simulink library "nsd"  (Simulink 8.1)
settings: Solver=ode1  StartTime=0.0  StopTime=Inf  FixedStep=0.001  RelTol=1e-3
PostLoadFcn:
  | , if any(exist('dsrtsu_mdlpostloadfcn', 'file') == [2, 3, 6]), try dsrtsu_mdlpostloadfcn('Execute', bdroot); catch fprintf('Error in PostLoadFcn (dsrtsu_mdlpostloadfcn) for model "%s":\n %s\n', bdroot, lasterr); end, end,
undefined symbols (not defined in the file or in its folder): KIFO_SameDirecSpeed_kph
libraries: hcu_lib x1
settings Model: DSRTSU_INTERNAL_RTI_VER=450  DSRTSU_INTERNAL_RTI_TYPE=rti1401  RTICANMMDATA=struct('GeneralSetupData',struct('modelroot','D:\ELN150201\Phase3\branches\Model_with_Distance_trigger\AdasDragon\software\sw_development\arch\app\ifo','generalsettings',struct('filesettings',struct('destfolder',struct('Name','RTICANMM_FILES','Check',1),'buildfolder',struct('Name','.','Check',1),'AbsDestfolder',struct('Name','D:\ELN150201\Phase3\branches\Model_with_Distance_trigger\AdasDragon\software\sw_development\arch\app\ifo\RTICANMM_FILES'),'AbsBuildfolder',struct('Name','D:\ELN150201\Phase3\branches\Model_with_Distance_trigger\AdasDragon\software\sw_development\arch\app\ifo'))),'options',struct('addpaths',1,'rmpaths',1,'addtrcexclusion',logical(1),'cannavigator',struct('checkmonitoring',0),'show_usrtrc',0,'use_usrtrc',0),'advanced',struct('options',[1 1 1 1 1 1 1 1 1 1 1 1 1 1 1 1 1 1 1 1 1 1 1 1 1 1 1 1 1 1 1 1 1 1 1 1 1 1 1 1 1 1 1 1 1 1 1 1 1 1 1 1 1 1 1 1 1 1 1 1 1 1 1 1 1 1 1 1 1 1 1 1 1 1 1 1 1 1 1 1 1 1 1 1 1 1 1 1 1 1 1 1 1 1 1 1 1 1 1 1]),'MPSetup',{{}},'modelname','nsd','block','nsd'))  DSRTSU_INTERNAL_RTIFPGA=40  Creator=tescamilla  LastModifiedBy=AT015555

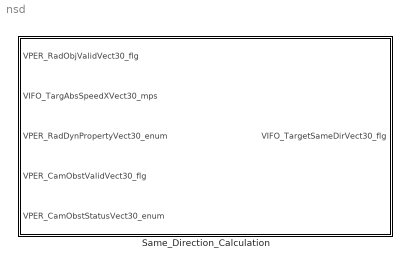
== system nsd ==
  Same_Direction_Calculation : Subsystem

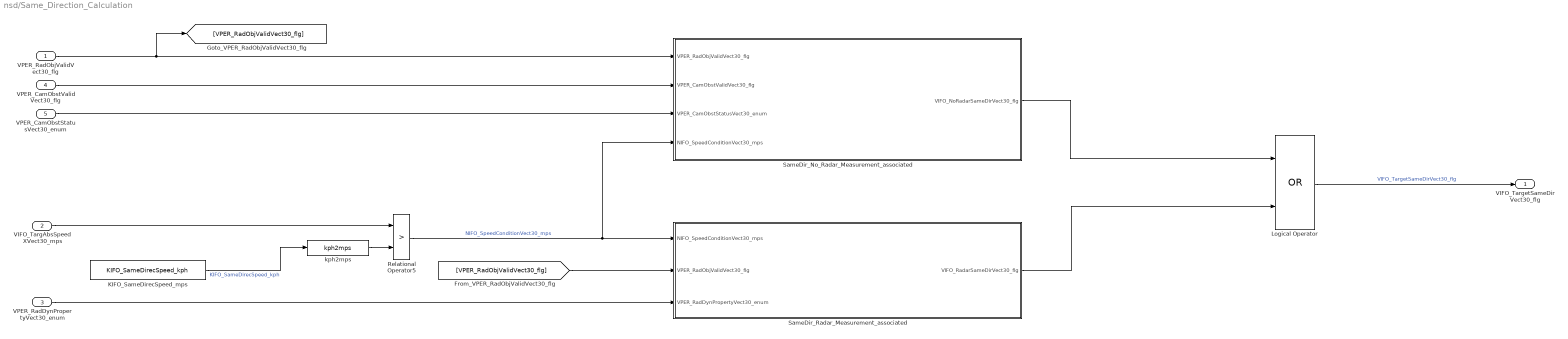
== system nsd/Same_Direction_Calculation ==
  VPER_RadObjValidVect30_flg : Inport
  VIFO_TargAbsSpeedXVect30_mps : Inport  Port=2
  VPER_RadDynPropertyVect30_enum : Inport  Port=3
  VPER_CamObstValidVect30_flg : Inport  Port=4
  VPER_CamObstStatusVect30_enum : Inport  Port=5
  KIFO_SameDirecSpeed_mps : Constant  Value=KIFO_SameDirecSpeed_kph  OutDataTypeStr=single
  Logical Operator : Logic  Operator=OR  AllPortsSameDT=off  OutDataTypeStr=boolean
  Relational Operator5 : RelationalOperator  Operator=>  OutDataTypeStr=boolean
  SameDir_No_Radar_Measurement_associated : Subsystem  TreatAsAtomicUnit=on
  SameDir_Radar_Measurement_associated : Subsystem  TreatAsAtomicUnit=on
  kph2mps : hcu_lib/kph2mps
  VIFO_TargetSameDirVect30_flg : Outport
  wires:
  Logical Operator/1 -> VIFO_TargetSameDirVect30_flg/1  "VIFO_TargetSameDirVect30_flg"
  VIFO_TargAbsSpeedXVect30_mps/1 -> Relational Operator5/1
  KIFO_SameDirecSpeed_mps/1 -> kph2mps/1  "KIFO_SameDirecSpeed_kph"
  kph2mps/1 -> Relational Operator5/2
  Relational Operator5/1 -> SameDir_No_Radar_Measurement_associated/4(NIFO_SpeedConditionVect30_mps), SameDir_Radar_Measurement_associated/1(NIFO_SpeedConditionVect30_mps)  "NIFO_SpeedConditionVect30_mps"
  SameDir_No_Radar_Measurement_associated/1(VIFO_NoRadarSameDirVect30_flg) -> Logical Operator/1
  SameDir_Radar_Measurement_associated/1(VIFO_RadarSameDirVect30_flg) -> Logical Operator/2
  VPER_RadObjValidVect30_flg/1 -> [VPER_RadObjValidVect30_flg], SameDir_No_Radar_Measurement_associated/1(VPER_RadObjValidVect30_flg)
  VPER_CamObstValidVect30_flg/1 -> SameDir_No_Radar_Measurement_associated/2(VPER_CamObstValidVect30_flg)
  VPER_CamObstStatusVect30_enum/1 -> SameDir_No_Radar_Measurement_associated/3(VPER_CamObstStatusVect30_enum)
  VPER_RadDynPropertyVect30_enum/1 -> SameDir_Radar_Measurement_associated/3(VPER_RadDynPropertyVect30_enum)
  [VPER_RadObjValidVect30_flg] -> SameDir_Radar_Measurement_associated/2(VPER_RadObjValidVect30_flg)

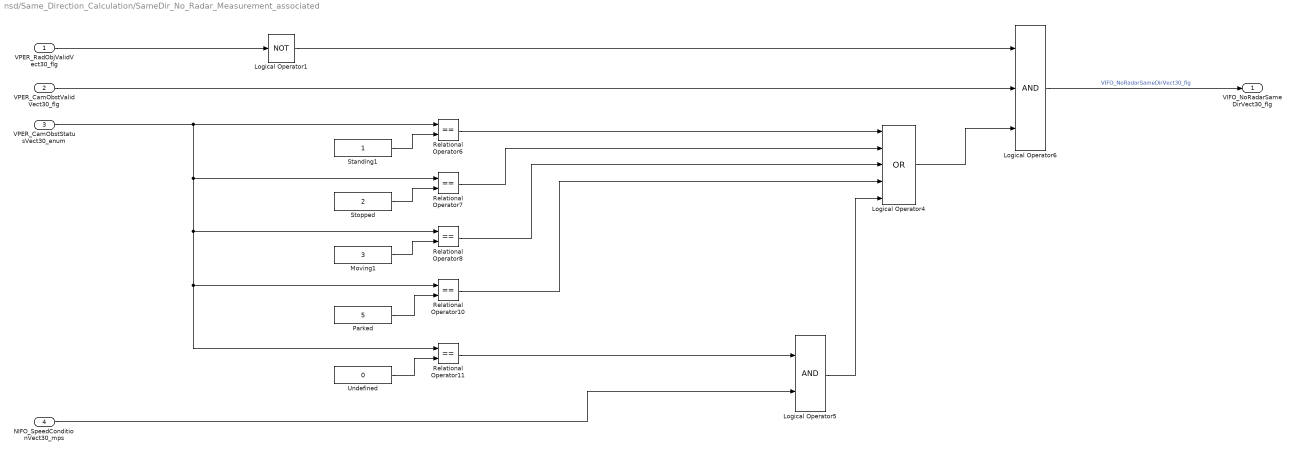
== system nsd/Same_Direction_Calculation/SameDir_No_Radar_Measurement_associated ==
  VPER_RadObjValidVect30_flg : Inport
  VPER_CamObstValidVect30_flg : Inport  Port=2
  VPER_CamObstStatusVect30_enum : Inport  Port=3
  NIFO_SpeedConditionVect30_mps : Inport  Port=4
  Logical Operator1 : Logic  Operator=NOT  AllPortsSameDT=off  OutDataTypeStr=boolean
  Logical Operator4 : Logic  Operator=OR  Inputs=5  AllPortsSameDT=off  OutDataTypeStr=boolean
  Logical Operator5 : Logic  AllPortsSameDT=off  OutDataTypeStr=boolean
  Logical Operator6 : Logic  Inputs=3  AllPortsSameDT=off  OutDataTypeStr=boolean
  Moving1 : Constant  Value=3
  Parked : Constant  Value=5
  Relational Operator{6..8,10..11} (5 alike) : RelationalOperator  Operator===  OutDataTypeStr=boolean
  Standing1 : Constant
  Stopped : Constant  Value=2
  Undefined : Constant  Value=0
  VIFO_NoRadarSameDirVect30_flg : Outport
  wires:
  Standing1/1 -> Relational Operator6/2
  Stopped/1 -> Relational Operator7/2
  Moving1/1 -> Relational Operator8/2
  Parked/1 -> Relational Operator10/2
  Relational Operator6/1 -> Logical Operator4/1
  Relational Operator7/1 -> Logical Operator4/2
  Relational Operator8/1 -> Logical Operator4/3
  Relational Operator10/1 -> Logical Operator4/4
  Undefined/1 -> Relational Operator11/2
  VPER_CamObstStatusVect30_enum/1 -> Relational Operator11/1, Relational Operator10/1, Relational Operator8/1, Relational Operator7/1, Relational Operator6/1
  Relational Operator11/1 -> Logical Operator5/1
  NIFO_SpeedConditionVect30_mps/1 -> Logical Operator5/2
  Logical Operator5/1 -> Logical Operator4/5
  VPER_CamObstValidVect30_flg/1 -> Logical Operator6/2
  Logical Operator4/1 -> Logical Operator6/3
  Logical Operator6/1 -> VIFO_NoRadarSameDirVect30_flg/1  "VIFO_NoRadarSameDirVect30_flg"
  VPER_RadObjValidVect30_flg/1 -> Logical Operator1/1
  Logical Operator1/1 -> Logical Operator6/1

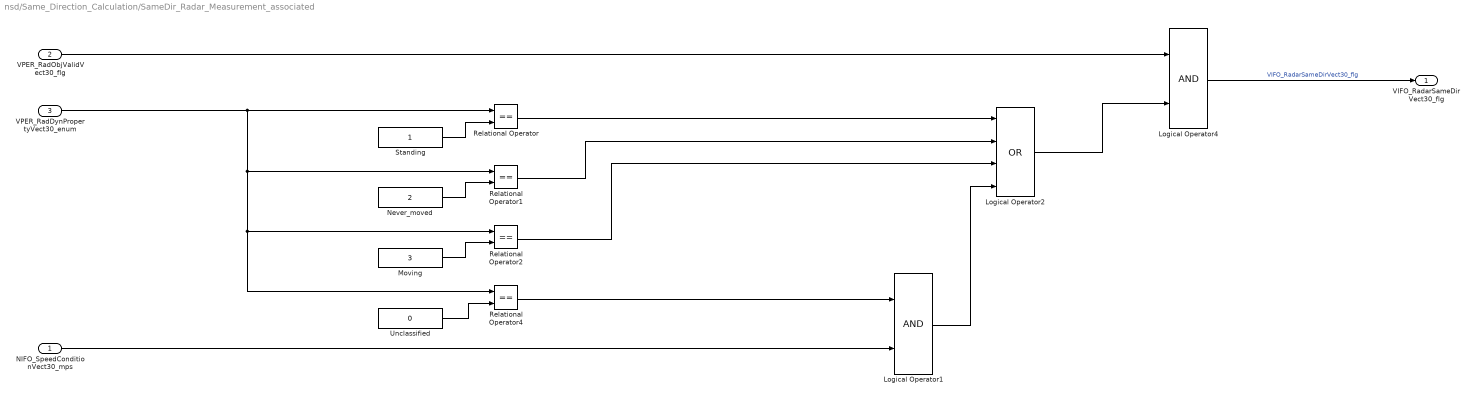
== system nsd/Same_Direction_Calculation/SameDir_Radar_Measurement_associated ==
  NIFO_SpeedConditionVect30_mps : Inport
  VPER_RadObjValidVect30_flg : Inport  Port=2
  VPER_RadDynPropertyVect30_enum : Inport  Port=3
  Logical Operator1 : Logic  AllPortsSameDT=off  OutDataTypeStr=boolean
  Logical Operator2 : Logic  Operator=OR  Inputs=4  AllPortsSameDT=off  OutDataTypeStr=boolean
  Logical Operator4 : Logic  AllPortsSameDT=off  OutDataTypeStr=boolean
  Moving : Constant  Value=3
  Never_moved : Constant  Value=2
  Relational Operator{,1..2,4} (4 alike) : RelationalOperator  Operator===  OutDataTypeStr=boolean
  Standing : Constant
  Unclassified : Constant  Value=0
  VIFO_RadarSameDirVect30_flg : Outport
  wires:
  Standing/1 -> Relational Operator/2
  Never_moved/1 -> Relational Operator1/2
  Moving/1 -> Relational Operator2/2
  Unclassified/1 -> Relational Operator4/2
  VPER_RadDynPropertyVect30_enum/1 -> Relational Operator4/1, Relational Operator2/1, Relational Operator1/1, Relational Operator/1
  Relational Operator/1 -> Logical Operator2/1
  Relational Operator1/1 -> Logical Operator2/2
  Relational Operator2/1 -> Logical Operator2/3
  Relational Operator4/1 -> Logical Operator1/1
  NIFO_SpeedConditionVect30_mps/1 -> Logical Operator1/2
  Logical Operator1/1 -> Logical Operator2/4
  Logical Operator2/1 -> Logical Operator4/2
  VPER_RadObjValidVect30_flg/1 -> Logical Operator4/1
  Logical Operator4/1 -> VIFO_RadarSameDirVect30_flg/1  "VIFO_RadarSameDirVect30_flg"
